simulink model "model1"  (R2024b)
settings: Solver=VariableStepAuto  StartTime=0.0  StopTime=10.0  RelTol=1e-3
undefined symbols (not defined in the file): A, Bw, C, Dw, L, Pival
libraries: simulink x4
settings Model: Creator=Mehmet  LastModifiedBy=Mehmet

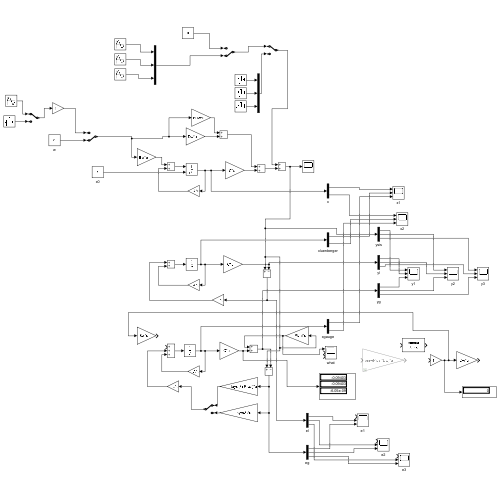
[thumbnail: Simulink's stored preview of the top-level diagram]
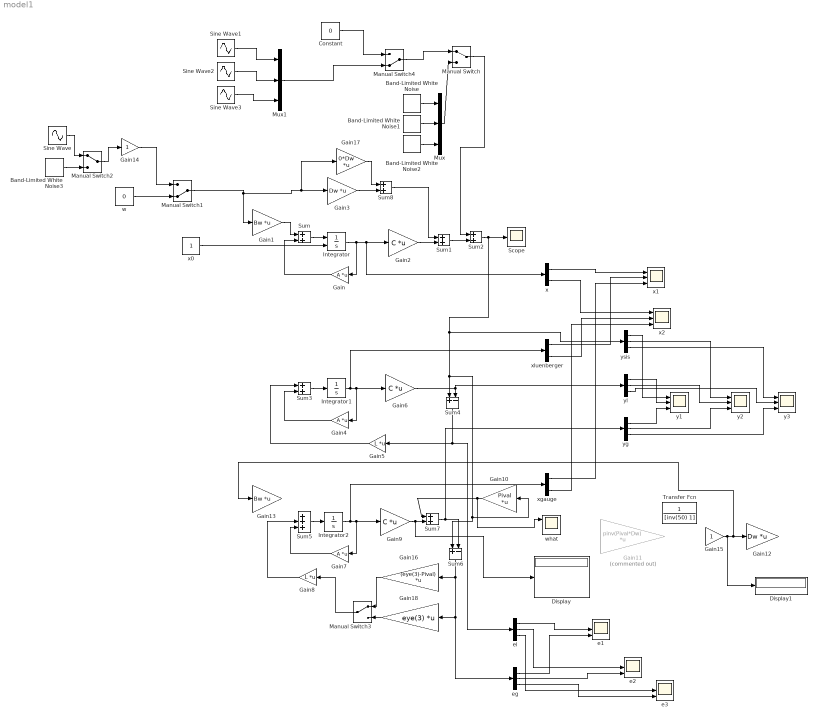
== system model1 ==
  Band-Limited White Noise : simulink/Sources/Band-Limited White Noise  Cov=[0.1]  Ts=0.1  seed=[23345]
  Band-Limited White Noise1 : simulink/Sources/Band-Limited White Noise  Cov=[0.01]  Ts=0.1  seed=[23343]
  Band-Limited White Noise2 : simulink/Sources/Band-Limited White Noise  Cov=[0.01]  Ts=0.1  seed=[23341]
  Band-Limited White Noise3 : simulink/Sources/Band-Limited White Noise  Cov=[0.01]  Ts=0.1  seed=[123]
  Constant : Constant  Value=0
  Display : Display
  Display1 : Display
  Gain : Gain  Gain=A  Multiplication=Matrix(K*u)
  Gain1 : Gain  Gain=Bw  Multiplication=Matrix(K*u)
  Gain10 : Gain  Gain=Pival  Multiplication=Matrix(K*u)
  Gain11 : Gain  Commented=on  Gain=pinv(Pival*Dw)  Multiplication=Matrix(K*u)
  Gain12 : Gain  Gain=Dw  Multiplication=Matrix(K*u)
  Gain13 : Gain  Gain=Bw  Multiplication=Matrix(K*u)
  Gain14 : Gain
  Gain15 : Gain
  Gain16 : Gain  Gain=(eye(3)-Pival)  Multiplication=Matrix(K*u)
  Gain17 : Gain  Gain=0*Dw  Multiplication=Matrix(K*u)
  Gain18 : Gain  Gain=eye(3)  Multiplication=Matrix(K*u)
  Gain2 : Gain  Gain=C  Multiplication=Matrix(K*u)
  Gain3 : Gain  Gain=Dw  Multiplication=Matrix(K*u)
  Gain4 : Gain  Gain=A  Multiplication=Matrix(K*u)
  Gain5 : Gain  Gain=L  Multiplication=Matrix(K*u)
  Gain6 : Gain  Gain=C  Multiplication=Matrix(K*u)
  Gain7 : Gain  Gain=A  Multiplication=Matrix(K*u)
  Gain8 : Gain  Gain=L  Multiplication=Matrix(K*u)
  Gain9 : Gain  Gain=C  Multiplication=Matrix(K*u)
  Integrator : Integrator  InitialConditionSource=external
  Integrator1 : Integrator
  Integrator2 : Integrator
  Manual Switch : ManualSwitch
  Manual Switch1 : ManualSwitch  CurrentSetting=0
  Manual Switch2 : ManualSwitch
  Manual Switch3 : ManualSwitch
  Manual Switch4 : ManualSwitch  CurrentSetting=0
  Mux : Mux  Inputs=3
  Mux1 : Mux  Inputs=3
  Scope : Scope
  Sine Wave : Sin  Frequency=10  SampleTime=0
  Sine Wave1 : Sin  Frequency=10  SampleTime=0
  Sine Wave2 : Sin  Frequency=20  SampleTime=0
  Sine Wave3 : Sin  Frequency=30  SampleTime=0
  Sum{,1..3,7..8} (6 alike) : Sum
  Sum4 : Sum  Inputs=+-
  Sum5 : Sum  Inputs=+++
  Sum6 : Sum  Inputs=+-
  Transfer Fcn : TransferFcn  Denominator=[inv(50) 1]
  e1 : Scope  NumInputPorts=3
  e2 : Scope  NumInputPorts=3
  e3 : Scope  NumInputPorts=3
  eg : Demux  Outputs=3
  el : Demux  Outputs=3
  w : Constant  Value=0
  what : Scope  NumInputPorts=3
  x : Demux  Outputs=2
  x0 : Constant
  x1 : Scope  NumInputPorts=3
  x2 : Scope  NumInputPorts=3
  xgauge : Demux  Outputs=2
  xluenberger : Demux  Outputs=2
  y1 : Scope  NumInputPorts=3
  y2 : Scope  NumInputPorts=3
  y3 : Scope  NumInputPorts=3
  yg : Demux  Outputs=3
  yl : Demux  Outputs=3
  ysis : Demux  Outputs=3
  wires:
  x0/1 -> Integrator/2
  Sum/1 -> Integrator/1
  Integrator/1 -> x/1, Gain2/1, Gain/1
  Gain/1 -> Sum/2
  Manual Switch1/1 -> Gain1/1, Gain17/1, Gain3/1
  Gain2/1 -> Sum1/2
  Sum8/1 -> Sum1/1
  Sum1/1 -> Sum2/2
  Band-Limited White Noise2/1 -> Mux/3
  Band-Limited White Noise1/1 -> Mux/2
  Band-Limited White Noise/1 -> Mux/1
  Manual Switch/1 -> Sum2/1
  Gain4/1 -> Sum3/2
  Gain6/1 -> yl/1, Sum4/2
  Sum3/1 -> Integrator1/1
  Integrator1/1 -> xluenberger/1, Gain6/1, Gain4/1
  Gain5/1 -> Sum3/1
  Sum4/1 -> Gain5/1, el/1
  x/1 -> x1/1
  xluenberger/1 -> x1/2
  x/2 -> x2/1
  xluenberger/2 -> x2/2
  Manual Switch4/1 -> Manual Switch/1
  Mux/1 -> Manual Switch/2
  Sum2/1 -> ysis/1, Gain10/1, Sum6/1, Sum4/1, Scope/1
  Gain8/1 -> Sum5/2
  Sum7/1 -> yg/1, Sum6/2
  Gain7/1 -> Sum5/3
  Integrator2/1 -> xgauge/1, Gain9/1, Gain7/1
  Sum5/1 -> Integrator2/1
  Gain9/1 -> Display/1, Sum7/2
  xgauge/1 -> x1/3
  xgauge/2 -> x2/3
  yl/1 -> y1/2
  yg/1 -> y1/3
  ysis/1 -> y1/1
  ysis/2 -> y2/1
  yl/2 -> y2/2
  yg/2 -> y2/3
  ysis/3 -> y3/1
  yl/3 -> y3/2
  yg/3 -> y3/3
  Sine Wave/1 -> Manual Switch2/1
  Gain14/1 -> Manual Switch1/1
  Gain15/1 -> Display1/1, Gain13/1, Gain12/1
  w/1 -> Manual Switch1/2
  Sum6/1 -> eg/1, Gain18/1, Gain16/1
  Gain16/1 -> Manual Switch3/1
  Band-Limited White Noise3/1 -> Manual Switch2/2
  Manual Switch2/1 -> Gain14/1
  Gain3/1 -> Sum8/2
  Gain17/1 -> Sum8/1
  Gain18/1 -> Manual Switch3/2
  Manual Switch3/1 -> Gain8/1
  el/1 -> e1/2
  eg/1 -> e1/3
  el/2 -> e2/2
  eg/2 -> e2/3
  el/3 -> e3/2
  eg/3 -> e3/3
  Gain1/1 -> Sum/1
  Gain10/1 -> what/1, Sum7/1
  Constant/1 -> Manual Switch4/1
  Mux1/1 -> Manual Switch4/2
  Sine Wave3/1 -> Mux1/3
  Sine Wave2/1 -> Mux1/2
  Sine Wave1/1 -> Mux1/1
